simulink model "lab1"  (R2017b)
settings: Solver=ode4  StartTime=0.0  StopTime=20  FixedStep=0.001  RelTol=1e-3
settings Model: Creator=ayushi  LastModifiedBy=ayushi

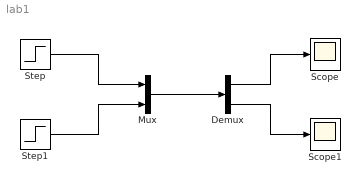
== system lab1 ==
  Demux : Demux  Outputs=2
  Mux : Mux  Inputs=2
  Scope : Scope
  Scope1 : Scope
  Step : Step  Time=0.5  After=0.5  SampleTime=0
  Step1 : Step  SampleTime=0
  wires:
  Step/1 -> Mux/1
  Step1/1 -> Mux/2
  Mux/1 -> Demux/1
  Demux/1 -> Scope/1
  Demux/2 -> Scope1/1
